simulink model "dcshuntwithspeed"  (R2024b)
settings: Solver=FixedStepDiscrete  StartTime=0.0  StopTime=10.0  RelTol=1e-3  EnableMultiTasking=on
libraries: c2802xlib x3
settings Model: SimulationMode=external  ExtModeTrigDuration=8  Creator=admin
settings SolverCC: AlgebraicLoopSolver=TrustRegion
settings DataIOCC: ReturnWorkspaceOutputs=off
settings OptimizationCC: DefaultUnderspecifiedDataType=single  PassReuseOutputArgsAs=Individual arguments  MaxStackSize=512  EfficientTunableParamExpr=on
settings DebuggingCC: ParameterTunabilityLossMsg=error  UnconnectedInputMsg=warning  UnconnectedOutputMsg=warning  UnconnectedLineMsg=warning  ArithmeticOperatorsInVariantConditions=warning
settings HardwareCC: ProdBitPerChar=16  ProdBitPerInt=16  ProdBitPerPointer=32  ProdBitPerSizeT=32  ProdBitPerPtrDiffT=32  ProdLargestAtomicInteger=Integer  ProdLargestAtomicFloat=None  ProdWordSize=16  ProdLongLongMode=on  ProdHWDeviceType=Texas Instruments->C2000
settings ModelReferenceCC: EnableRefExpFcnMdlSchedulingChecks=on
settings SFSimCC: SimUseLocalCustomCode=off  MATLABDynamicMemAlloc=off  CustomCodeUndefinedFunction=UseInterfaceOnly
settings RTWCC: Description=Embedded Coder  SystemTargetFile=ert.tlc  HardwareBoard=TI Piccolo F2802x  TemplateMakefile=ert_default_tmf  GenerateReport=on  RTWUseLocalCustomCode=off  Toolchain=Texas Instruments Code Composer Studio (C2000)  IncludeHyperlinkInReport=on  LaunchReport=on  GenerateTraceInfo=on  GenerateTraceReport=on  GenerateTraceReportSl=on  GenerateTraceReportSf=on  GenerateTraceReportEml=on  GPUComputeCapability=3.5
settings CodeAppCC: ForceParamTrailComments=on  IgnoreCustomStorageClasses=off  OperatorAnnotations=on  SimulinkDataObjDesc=on  SFDataObjDesc=on  MATLABFcnDesc=on  InsertBlockDesc=on  StateflowObjectComments=on  MATLABSourceComments=on
settings ERTTargetCC: CodeReplacementLibrary=TI C28x  SupportContinuousTime=on  ExtMode=on  ExtModeTransport=3  ExtModeMexArgs='127.0.0.1' 0 17725  InlinedParameterPlacement=Hierarchical  DynamicArrayContainerType=coder::array

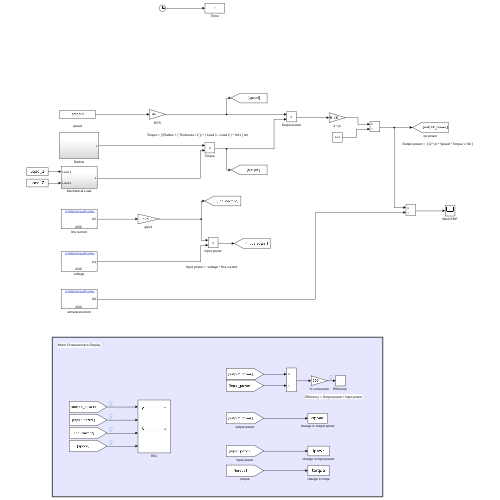
[thumbnail: Simulink's stored preview of the top-level diagram]
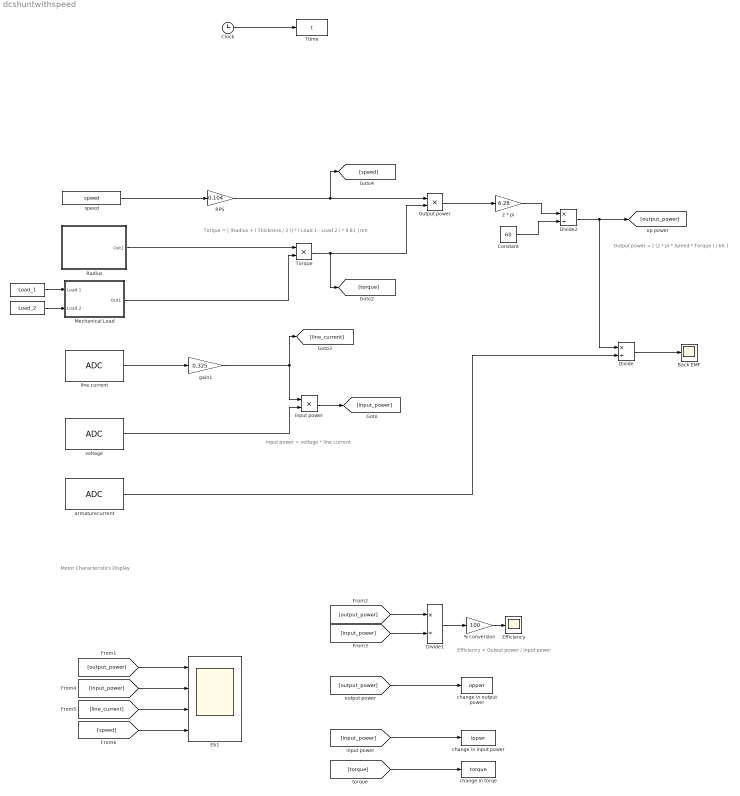
== system dcshuntwithspeed ==
  note: Efficiency = Output power / Input power
  note: Input power = voltage * line current
  note: Output power = [ (2 * pi * Speed * Torque ) / 60 ]
  note: Torque = [ (Radius + ( Thickness / 2 )) * ( Load 1 - Load 2 ) * 9.81 ] nm
  note: Motor Characteristics Display
  " " : FromWorkspace  VariableName=Load_1
  " speed" : FromWorkspace  VariableName=speed
  "  " : FromWorkspace  VariableName=Load_2
  % conversion : Gain  Gain=100
  2 * pi : Gain  Gain=6.28
  Back EMF : Scope
  Clock : Clock
  Constant : Constant  Value=60
  Divide : Product  Inputs=*/
  Divide1 : Product  Inputs=*/
  Divide2 : Product  Inputs=*/
  Eb1 : Scope  NumInputPorts=4
  "Efficiency " : Scope
  Input power : Product
  Mechanical Load : Subsystem
  Output power : Product
  RPS : Gain  Gain=0.104
  Radius : Subsystem
  Torque : Product
  Ttime : ToWorkspace  VariableName=t  SampleTime=-1
  armaturecurrent : c2802xlib/ADC  blkParamProc=C2000  ADCModule=1  samplingMode=Single sample mode  ADCResolution=12-bit (Single-ended input)  useSOC1=SOC0  useSOC2=SOC0_SOC1  SOCAcquisitionWindow=7  SOCTriggerSource=Software  SOCInterruptTrigger=No ADCINT  Ts=0.001  dType=uint16  postInterrupt=off  interruptSel=ADCINT1  ADCINTContinuous=on  endma=off  chdma=1  conv1=ADCINA0  conv2=ADCINA0 and ADCINB0  conv1_Type4=ADCIN0  conv2_Type4=ADCIN0 and ADCIN1
  "change in input power " : ToWorkspace  VariableName=ippwr  SampleTime=-1
  change in output power : ToWorkspace  VariableName=oppwr  SampleTime=-1
  change in torqe : ToWorkspace  VariableName=torque  SampleTime=-1
  gain1 : Gain  Gain=0.325
  "line current " : c2802xlib/ADC  blkParamProc=C2000  ADCModule=1  samplingMode=Single sample mode  ADCResolution=12-bit (Single-ended input)  useSOC1=SOC2  useSOC2=SOC0_SOC1  SOCAcquisitionWindow=7  SOCTriggerSource=Software  SOCInterruptTrigger=No ADCINT  Ts=0.001  dType=double  postInterrupt=off  interruptSel=ADCINT1  ADCINTContinuous=on  endma=off  chdma=1  conv1=ADCINA2  conv2=ADCINA0 and ADCINB0  conv1_Type4=ADCIN0  conv2_Type4=ADCIN0 and ADCIN1
  voltage : c2802xlib/ADC  blkParamProc=C2000  ADCModule=1  samplingMode=Single sample mode  ADCResolution=12-bit (Single-ended input)  useSOC1=SOC1  useSOC2=SOC0_SOC1  SOCAcquisitionWindow=7  SOCTriggerSource=Software  SOCInterruptTrigger=No ADCINT  Ts=0.001  dType=double  postInterrupt=off  interruptSel=ADCINT1  ADCINTContinuous=on  endma=off  chdma=1  conv1=ADCINA1  conv2=ADCINA0 and ADCINB0  conv1_Type4=ADCIN0  conv2_Type4=ADCIN0 and ADCIN1
  wires:
  Torque/1 -> [torque], Output power/2
  gain1/1 -> [line_current], Input power/1
  " speed"/1 -> RPS/1
  Clock/1 -> Ttime/1
  "line current "/1 -> gain1/1
  RPS/1 -> [speed], Output power/1
  Output power/1 -> 2 * pi/1
  armaturecurrent/1 -> Divide/2
  Divide/1 -> Back EMF/1
  voltage/1 -> Input power/2
  Mechanical Load/1(Out1) -> Torque/2
  " "/1 -> Mechanical Load/1(Load 1)
  "  "/1 -> Mechanical Load/2(Load 2)
  Radius/1(Out1) -> Torque/1
  Input power/1 -> [input_power]
  [input_power] -> "change in input power "/1
  [output_power] -> change in output power/1
  [output_power] -> Divide1/1
  [input_power] -> Divide1/2
  [torque] -> change in torqe/1
  [output_power] -> Eb1/1
  [input_power] -> Eb1/2
  [line_current] -> Eb1/3
  [speed] -> Eb1/4
  2 * pi/1 -> Divide2/1
  Constant/1 -> Divide2/2
  Divide2/1 -> Divide/1, [output_power]
  % conversion/1 -> "Efficiency "/1
  Divide1/1 -> % conversion/1

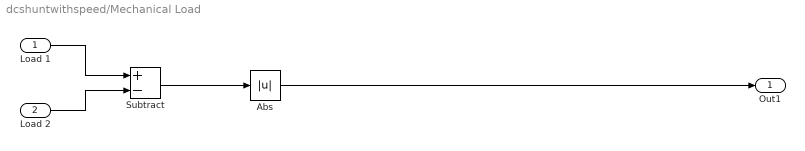
== system dcshuntwithspeed/Mechanical Load ==
  Load 1 : Inport
  Load 2 : Inport  Port=2
  Abs : Abs  SaturateOnIntegerOverflow=off
  Subtract : Sum  Inputs=+-
  Out1 : Outport
  wires:
  Load 1/1 -> Subtract/1
  Load 2/1 -> Subtract/2
  Abs/1 -> Out1/1
  Subtract/1 -> Abs/1

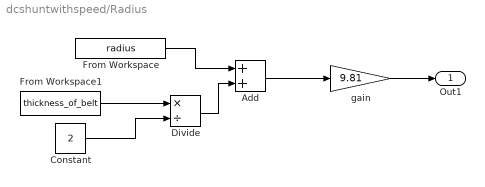
== system dcshuntwithspeed/Radius ==
  Add : Sum
  Constant : Constant  Value=2
  Divide : Product  Inputs=*/
  From Workspace : FromWorkspace  VariableName=radius  SampleTime=-1
  From Workspace1 : FromWorkspace  VariableName=thickness_of_belt  SampleTime=-1
  gain : Gain  Gain=9.81
  Out1 : Outport
  wires:
  From Workspace/1 -> Add/1
  Add/1 -> gain/1
  gain/1 -> Out1/1
  From Workspace1/1 -> Divide/1
  Divide/1 -> Add/2
  Constant/1 -> Divide/2
